simulink model "MSIP_Speed_Control_abc1a_84"  (R2025a)
settings: Solver=FixedStepAuto  StartTime=0.0  StopTime=150  FixedStep=1e-4  MaxStep=1e-3  RelTol=1e-3
model workspace (MAT data in the model file):
  Freq = 60
values from neighbouring files (symbols this model uses):
  b_MS = 1e-3    (= 0.001)    [data_MSIP_julio2025.m]
  beta_d_MS = pd_MS    (= 40)    [data_MSIP_julio2025.m]
  gamq = 2*J_MS*Lq_MS/(3*np_MS*lambda_MS)    (= 0.00452625826005)    [data_MSIP_julio2025.m]
  J_MS = 1e-1    (= 0.1)    [data_MSIP_julio2025.m]
  lambda_MS = 67.09e-2    (= 0.6709)    [data_MSIP_julio2025.m]
  Ld_MS = 22.1e-3    (= 0.0221)    [data_MSIP_julio2025.m]
  Lq_MS = 91.1e-3    (= 0.0911)    [data_MSIP_julio2025.m]
  np_MS = 2    [data_MSIP_julio2025.m]
  Rs_MS = 6.51e-1    (= 0.651)    [data_MSIP_julio2025.m]
undefined symbols (not defined in the file or in its folder): plecs
libraries: plecslib_extras2 x3, spsRMSLib x2, spsPLL3phLib x1, nesl_utility x1, spsTHDLib x1
(part 1 of 2)
settings Model: SimulationMode=accelerator  PauseTimes=0.01  Creator=RUBEN TAPIA OLVERA  LastModifiedBy=avalder
settings SolverCC: AlgebraicLoopSolver=TrustRegion
settings DataIOCC: ReturnWorkspaceOutputs=off
settings OptimizationCC: LifeSpan=inf
settings DebuggingCC: MaxConsecutiveZCsMsg=none  UnconnectedInputMsg=warning  UnconnectedOutputMsg=warning  UnconnectedLineMsg=warning  SFUnexpectedBacktrackingDiag=warning  SFNoUnconditionalDefaultTransitionDiag=warning  SFExecutionAtInitializationDiag=none  ArithmeticOperatorsInVariantConditions=warning
settings ModelReferenceCC: EnableRefExpFcnMdlSchedulingChecks=on
settings SFSimCC: SimUseLocalCustomCode=off  CustomCodeUndefinedFunction=UseInterfaceOnly
settings RTWCC: RTWUseLocalCustomCode=off  GPUComputeCapability=3.5
settings CodeAppCC: StateflowObjectComments=on
settings GRTTargetCC: TargetLangStandard=C89/C90 (ANSI)
settings ConfigComp: CovMetricSettings=dw  CovSaveCumulativeToWorkspaceVar=on  CovSaveSingleToWorkspaceVar=on  CovExternalEMLEnable=off
settings SimscapeCC: SimscapeNormalizeSystem=off

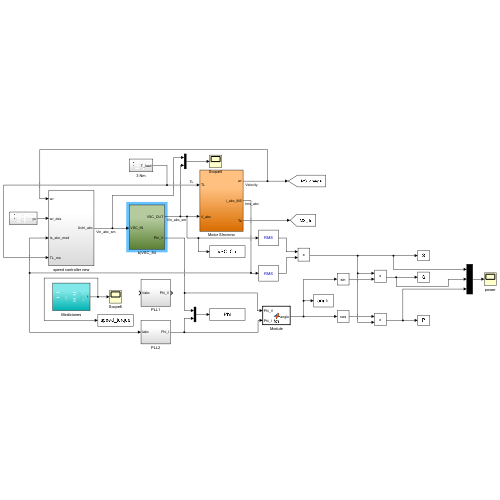
[thumbnail: Simulink's stored preview of the top-level diagram]
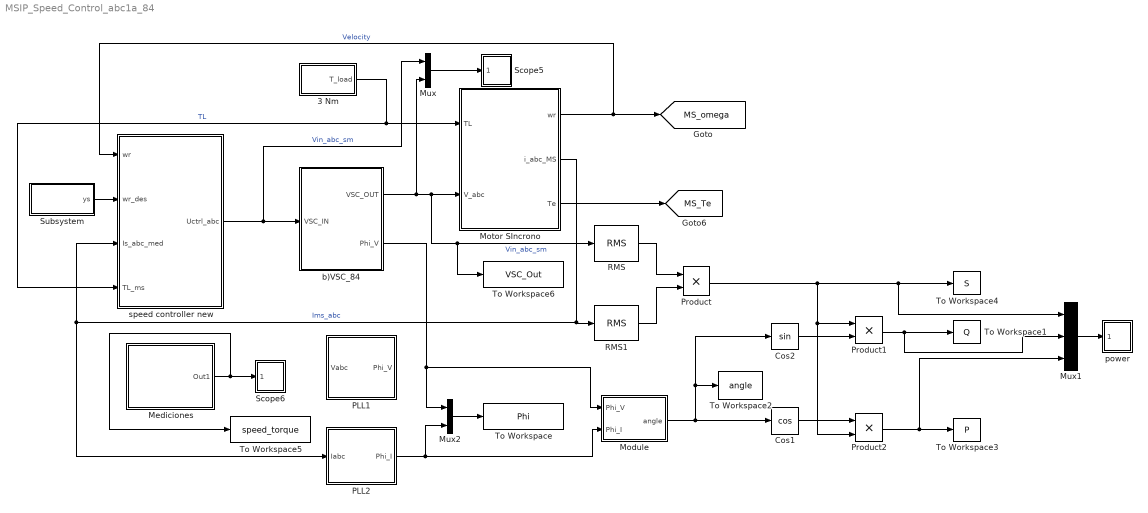
== system MSIP_Speed_Control_abc1a_84 ==
  3 Nm : Subsystem
  Cos1 : Trigonometry  Operator=cos
  Cos2 : Trigonometry
  Mediciones : Subsystem
  Module : MATLAB Function  TreatAsAtomicUnit=on
  Motor SIncrono : Subsystem
  Mux : Mux  Inputs=2
  Mux1 : Mux  Inputs=3
  Mux2 : Mux  Inputs=2
  PLL1 : Subsystem
  PLL2 : Subsystem
  Product : Product
  Product1 : Product
  Product2 : Product
  RMS : spsRMSLib/RMS  TrueRMS=on  Freq=Freq  RMSInit=0  Ts=0
  RMS1 : spsRMSLib/RMS  TrueRMS=on  Freq=Freq  RMSInit=0  Ts=0
  Scope5 : Subsystem  LoadFcn=plecs('sl', 300);  InitFcn=plecs('sl', 314);  StartFcn=plecs('sl', 308);  StopFcn=plecs('sl', 309);  mask{Settings=<binary blob, 776 chars, not shown>}
      mask init:
      | plecs('sl', 315);
      settings: CopyFcn=plecs('sl', 303);  DeleteFcn=plecs('sl', 305);  UndoDeleteFcn=plecs('sl', 306);  PreSaveFcn=plecs('sl', 311);  NameChangeFcn=plecs('sl', 310);  DestroyFcn=plecs('sl', 307);  OpenFcn=plecs('sl', 302);  ErrorFcn=plerrorfcn
      mask Display: plot([0.1 0.9 0.9 0.1 0.1], [0.9 0.9 0.5 0.5 0.9])
  Scope6 : Subsystem  LoadFcn=plecs('sl', 300);  InitFcn=plecs('sl', 314);  StartFcn=plecs('sl', 308);  StopFcn=plecs('sl', 309);  mask{Settings=<binary blob, 752 chars, not shown>}
      mask init:
      | plecs('sl', 315);
      settings: CopyFcn=plecs('sl', 303);  DeleteFcn=plecs('sl', 305);  UndoDeleteFcn=plecs('sl', 306);  PreSaveFcn=plecs('sl', 311);  NameChangeFcn=plecs('sl', 310);  DestroyFcn=plecs('sl', 307);  OpenFcn=plecs('sl', 302);  ErrorFcn=plerrorfcn
      mask Display: plot([0.1 0.9 0.9 0.1 0.1], [0.9 0.9 0.5 0.5 0.9])
  Subsystem : Subsystem
  To Workspace : ToWorkspace  VariableName=Phi  SaveFormat=Timeseries  SampleTime=-1
  To Workspace1 : ToWorkspace  VariableName=Q  SaveFormat=Timeseries  SampleTime=-1
  To Workspace2 : ToWorkspace  VariableName=angle  SaveFormat=Timeseries  SampleTime=-1
  To Workspace3 : ToWorkspace  VariableName=P  SaveFormat=Timeseries  SampleTime=-1
  To Workspace4 : ToWorkspace  VariableName=S  SaveFormat=Timeseries  SampleTime=-1
  To Workspace5 : ToWorkspace  VariableName=speed_torque  SaveFormat=Timeseries  SampleTime=-1
  To Workspace6 : ToWorkspace  VariableName=VSC_Out  SaveFormat=Timeseries  SampleTime=-1
  b)VSC_84 : Subsystem
  power : Subsystem  LoadFcn=plecs('sl', 300);  InitFcn=plecs('sl', 314);  StartFcn=plecs('sl', 308);  StopFcn=plecs('sl', 309);  mask{Settings=<binary blob, 756 chars, not shown>}
      mask init:
      | plecs('sl', 315);
      settings: CopyFcn=plecs('sl', 303);  DeleteFcn=plecs('sl', 305);  UndoDeleteFcn=plecs('sl', 306);  PreSaveFcn=plecs('sl', 311);  NameChangeFcn=plecs('sl', 310);  DestroyFcn=plecs('sl', 307);  OpenFcn=plecs('sl', 302);  ErrorFcn=plerrorfcn
      mask Display: plot([0.1 0.9 0.9 0.1 0.1], [0.9 0.9 0.5 0.5 0.9])
  speed controller new : Subsystem
  tag scope: MS_Te=global, MS_omega=global
  wires:
  Motor SIncrono/1(wr) -> speed controller new/1(wr), [MS_omega]  "Velocity"
  3 Nm/1(T_load) -> speed controller new/4(TL_ms), Motor SIncrono/1(TL)  "TL"
  Motor SIncrono/3(Te) -> [MS_Te]
  Motor SIncrono/2(i_abc_MS) -> RMS1/1, speed controller new/3(Is_abc_med), PLL2/1(Iabc)  "Ims_abc"
  Subsystem/1(ys) -> speed controller new/2(wr_des)
  Mux2/1 -> To Workspace/1
  Module/1(angle) -> Cos1/1, To Workspace2/1, Cos2/1
  b)VSC_84/1(VSC_OUT) -> Mux/2, Motor SIncrono/2(V_abc), To Workspace6/1, RMS/1  "Vin_abc_sm"
  b)VSC_84/2(Phi_V) -> Mux2/1, Module/1(Phi_V)
  PLL2/1(Phi_I) -> Module/2(Phi_I), Mux2/2
  speed controller new/1(Uctrl_abc) -> b)VSC_84/1(VSC_IN), Mux/1  "Vin_abc_sm"
  Product/1 -> Product2/2, Product1/1, Mux1/1, To Workspace4/1
  RMS/1 -> Product/1
  RMS1/1 -> Product/2
  Mux/1 -> Scope5/1(1)
  Mediciones/1(Out1) -> To Workspace5/1, Scope6/1(1)
  Cos2/1 -> Product1/2
  Cos1/1 -> Product2/1
  Product1/1 -> Mux1/2, To Workspace1/1
  Product2/1 -> Mux1/3, To Workspace3/1
  Mux1/1 -> power/1(1)

== system MSIP_Speed_Control_abc1a_84/3 Nm ==
  Add : Sum  Inputs=+++
  TL1 : MATLAB Function  TreatAsAtomicUnit=on
  TL2 : MATLAB Function  TreatAsAtomicUnit=on
  TL3 : MATLAB Function  TreatAsAtomicUnit=on
  Tiempo1 : Clock
  T_load : Outport
  tag scope: TL_MS=global
  wires:
  Tiempo1/1 -> TL3/1(t), TL2/1(t), TL1/1(t)
  TL3/1(T_load3) -> Add/3
  TL1/1(T_load) -> Add/1
  TL2/1(T_load2) -> Add/2
  Add/1 -> T_load/1, [TL_MS]

== system MSIP_Speed_Control_abc1a_84/Mediciones ==
  Demux : Demux  Outputs=2
  Mux : Mux  Inputs=2
  Mux1 : Mux  Inputs=2
  Mux2 : Mux  Inputs=2
  Scope{1,3..6} (5 alike) : Scope
      Scope1 settings: Title=Currents  ActiveDisplayYMinimum=-0.00105  ActiveDisplayYMaximum=0.01123  DataLoggingVariableName=ScopeData3
      Scope3 settings: ActiveDisplayYMinimum=-1  ActiveDisplayYMaximum=1
      Scope4 settings: ActiveDisplayYMinimum=-1  ActiveDisplayYMaximum=1  DataLoggingVariableName=ScopeData4
      Scope5 settings: Title=Currents  ActiveDisplayYMinimum=-0.003  ActiveDisplayYMaximum=0.00033
      Scope6 settings: ActiveDisplayYMinimum=-23.57031  ActiveDisplayYMaximum=212.1328
  Out1 : Outport
  wires:
  [MS_omega] -> Scope3/1
  [TL_MS] -> Mux2/1  "MI_TL"
  Mux2/1 -> Mux/2, Scope4/1
  [MS_Te] -> Mux2/2  "MI_Te"
  [Idq_MS] -> Demux/1
  Demux/1 -> Scope1/1
  Demux/2 -> Scope5/1
  [MS_omega] -> Mux1/2  "w"
  [MSIP_w_des] -> Mux1/1  "w_req"
  Mux1/1 -> Mux/1, Scope6/1
  Mux/1 -> Out1/1

== system MSIP_Speed_Control_abc1a_84/Motor SIncrono ==
  TL : Inport
  V_abc : Inport  Port=2
  Clock : Clock
  Clock1 : Clock
  Demux : Demux  Outputs=2
  Electrical Subsystem : Subsystem
  Mechanical Subsystem : Subsystem
  Mux2 : Mux  Inputs=2
  abc/dq : Subsystem
  dq/abc : Subsystem
  wr : Outport
  i_abc_MS : Outport  Port=2
  Te : Outport  Port=3
  tag scope: Idq_MS=global
  wires:
  Mechanical Subsystem/1(wr_MS) -> wr/1, Electrical Subsystem/1(w)
  TL/1 -> Mechanical Subsystem/1(TL)
  Mechanical Subsystem/2(Te_MS) -> Te/1
  Demux/1 -> Electrical Subsystem/2(U_d_MS)
  Demux/2 -> Electrical Subsystem/3(U_q_MS)
  Electrical Subsystem/1(id_MS) -> Mux2/1, Mechanical Subsystem/2(i_d_MS)  "id"
  Electrical Subsystem/2(iq_MS) -> Mechanical Subsystem/3(i_q_MS), Mux2/2  "iq"
  Mux2/1 -> dq/abc/2(Ud_m), [Idq_MS]  "i_dq"
  Clock/1 -> dq/abc/1(t)
  dq/abc/1(Uabc_m) -> i_abc_MS/1  "abc"
  Clock1/1 -> abc/dq/1(t)
  abc/dq/1(Udq_m) -> Demux/1  "a"
  V_abc/1 -> abc/dq/2(Uabc_m)

== system MSIP_Speed_Control_abc1a_84/PLL1 ==
  Vabc : Inport
  3ph->SRF : plecslib_extras2/Transformations/3ph->SRF
      settings: SourceProductName=PLECS Extras
  Constant1 : Constant  Value=pi/2
  Demux : Demux  Outputs=2
  Divide : Product  Inputs=/*
  Kp1 : Gain  Gain=-1  SaturateOnIntegerOverflow=on  OutDataTypeStr=Inherit: Same as input  ParamDataTypeStr=Inherit: Same as input
  Kp2 : Gain  Gain=2  SaturateOnIntegerOverflow=on  OutDataTypeStr=Inherit: Same as input  ParamDataTypeStr=Inherit: Same as input
  Module : MATLAB Function  TreatAsAtomicUnit=on
  Sum2 : Sum  Inputs=|+-
  Sum3 : Sum  Inputs=|++
  Trigonometric Function2 : Trigonometry  Operator=atan
  Phi_V : Outport
  wires:
  Demux/2 -> Divide/2
  Vabc/1 -> 3ph->SRF/1
  Demux/1 -> Sum2/2
  Sum2/1 -> Divide/1
  Divide/1 -> Trigonometric Function2/1
  Sum3/1 -> Kp2/1
  Module/1(y) -> Sum2/1
  Kp2/1 -> Phi_V/1
  Trigonometric Function2/1 -> Kp1/1
  Kp1/1 -> Sum3/1
  Constant1/1 -> Sum3/2
  3ph->SRF/1 -> Demux/1, Module/1(u)

== system MSIP_Speed_Control_abc1a_84/PLL2 ==
  Iabc : Inport
  3ph->SRF : plecslib_extras2/Transformations/3ph->SRF
      settings: SourceProductName=PLECS Extras
  Constant1 : Constant  Value=pi/2
  Demux : Demux  Outputs=2
  Divide : Product  Inputs=/*
  Kp1 : Gain  Gain=-1  SaturateOnIntegerOverflow=on  OutDataTypeStr=Inherit: Same as input  ParamDataTypeStr=Inherit: Same as input
  Kp2 : Gain  Gain=2  SaturateOnIntegerOverflow=on  OutDataTypeStr=Inherit: Same as input  ParamDataTypeStr=Inherit: Same as input
  Module : MATLAB Function  TreatAsAtomicUnit=on
  Sum2 : Sum  Inputs=|+-
  Sum3 : Sum  Inputs=|++
  Trigonometric Function2 : Trigonometry  Operator=atan
  Phi_I : Outport
  wires:
  Demux/2 -> Divide/2
  Iabc/1 -> 3ph->SRF/1
  Demux/1 -> Sum2/2
  Sum2/1 -> Divide/1
  Divide/1 -> Trigonometric Function2/1
  Sum3/1 -> Kp2/1
  Module/1(y) -> Sum2/1
  Kp2/1 -> Phi_I/1
  Trigonometric Function2/1 -> Kp1/1
  Kp1/1 -> Sum3/1
  Constant1/1 -> Sum3/2
  3ph->SRF/1 -> Demux/1, Module/1(u)

== system MSIP_Speed_Control_abc1a_84/Scope5 ==
  1 : Inport
  " InputMux " : Subsystem
      mask Display: disp('Mux')
  " S-Function " : S-Function  FunctionName=plecs  SFunctionDeploymentMode=off  EnableBusSupport=off
  wires:
  1/1 -> " InputMux "/1(In1)
  " InputMux "/1(Out) -> " S-Function "/1

== system MSIP_Speed_Control_abc1a_84/Scope6 ==
  1 : Inport
  " InputMux " : Subsystem
      mask Display: disp('Mux')
  " S-Function " : S-Function  FunctionName=plecs  SFunctionDeploymentMode=off  EnableBusSupport=off
  wires:
  1/1 -> " InputMux "/1(In1)
  " InputMux "/1(Out) -> " S-Function "/1

== system MSIP_Speed_Control_abc1a_84/Subsystem ==
  Add : Sum  Inputs=+++
  Theta_Deseada : MATLAB Function  TreatAsAtomicUnit=on
  Theta_Deseada1 : MATLAB Function  TreatAsAtomicUnit=on
  Theta_Deseada2 : MATLAB Function  TreatAsAtomicUnit=on
  Tiempo1 : Clock
  ys : Outport
  tag scope: MSIP_w_des=global
  wires:
  Tiempo1/1 -> Theta_Deseada1/1(t), Theta_Deseada2/1(t), Theta_Deseada/1(t)
  Theta_Deseada/1(ys) -> Add/1
  Theta_Deseada1/1(ys) -> Add/2
  Theta_Deseada2/1(ys) -> Add/3
  Add/1 -> ys/1, [MSIP_w_des]

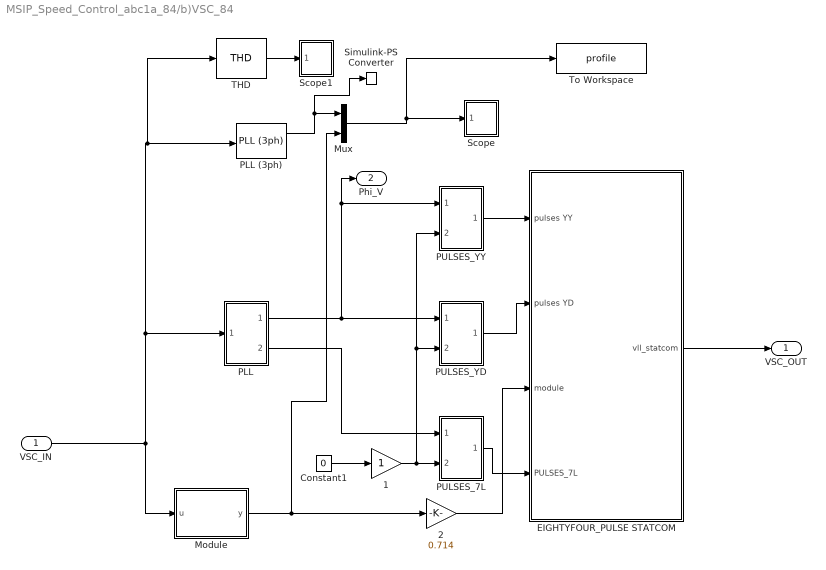
== system MSIP_Speed_Control_abc1a_84/b)VSC_84 ==
  VSC_IN : Inport
  1 : Gain  SaturateOnIntegerOverflow=on  OutDataTypeStr=Inherit: Same as input  ParamDataTypeStr=Inherit: Same as input
  2 : Gain  Gain=0.714  SaturateOnIntegerOverflow=on  OutDataTypeStr=Inherit: Same as input  ParamDataTypeStr=Inherit: Same as input
  Constant1 : Constant  Value=0
  EIGHTYFOUR_PULSE STATCOM : Subsystem  LoadFcn=plecs('sl', 200);  InitFcn=plecs('sl', 214);  StartFcn=plecs('sl', 208);  StopFcn=plecs('sl', 209);  mask(PlecsCircuit){PLECSData=<binary blob, 7880 chars, not shown>}
      mask prompts: PLECSData "PLECS Data (Do not delete or modify!)"
      mask help: Drag this block into a Simulink model to create a new electrical circuit.
      mask init:
      | % PLACE CUSTOM INITIALIZATIONS ABOVE
      | % DO NOT REMOVE
      | plecs('sl', 215);
      | % DO NOT REMOVE
      settings: CopyFcn=plecs('sl', 203);  DeleteFcn=plecs('sl', 205);  UndoDeleteFcn=plecs('sl', 206);  PreSaveFcn=plecs('sl', 211);  PostSaveFcn=plecs('sl', 201);  NameChangeFcn=plecs('sl', 210);  DestroyFcn=plecs('sl', 207);  PreCopyFcn=plecs('sl', 216);  OpenFcn=plecs('sl', 202);  ErrorFcn=plerrorfcn
      mask Display: disp('PLECS\nCircuit')
  Module : MATLAB Function  TreatAsAtomicUnit=on
  Mux : Mux  Inputs=2
  PLL : Subsystem
  PLL (3ph) : spsPLL3phLib/PLL (3ph)  Fmin=45  Par_Init=[0, 60]  ParK=[180, 3200, 1]  TcD=1e-4  MaxRateChangeFreq=12  FilterCutOffFreq=25  Ts=0  AGC=on
  PULSES_7L : Subsystem
  PULSES_YD : Subsystem
  PULSES_YY : Subsystem
  Scope : Subsystem  LoadFcn=plecs('sl', 300);  InitFcn=plecs('sl', 314);  StartFcn=plecs('sl', 308);  StopFcn=plecs('sl', 309);  mask{Settings=<binary blob, 752 chars, not shown>}
      mask init:
      | plecs('sl', 315);
      settings: CopyFcn=plecs('sl', 303);  DeleteFcn=plecs('sl', 305);  UndoDeleteFcn=plecs('sl', 306);  PreSaveFcn=plecs('sl', 311);  NameChangeFcn=plecs('sl', 310);  DestroyFcn=plecs('sl', 307);  OpenFcn=plecs('sl', 302);  ErrorFcn=plerrorfcn
      mask Display: plot([0.1 0.9 0.9 0.1 0.1], [0.9 0.9 0.5 0.5 0.9])
  Scope1 : Subsystem  LoadFcn=plecs('sl', 300);  InitFcn=plecs('sl', 314);  StartFcn=plecs('sl', 308);  StopFcn=plecs('sl', 309);  mask{Settings=<binary blob, 752 chars, not shown>}
      mask init:
      | plecs('sl', 315);
      settings: CopyFcn=plecs('sl', 303);  DeleteFcn=plecs('sl', 305);  UndoDeleteFcn=plecs('sl', 306);  PreSaveFcn=plecs('sl', 311);  NameChangeFcn=plecs('sl', 310);  DestroyFcn=plecs('sl', 307);  OpenFcn=plecs('sl', 302);  ErrorFcn=plerrorfcn
      mask Display: plot([0.1 0.9 0.9 0.1 0.1], [0.9 0.9 0.5 0.5 0.9])
  Simulink-PS Converter : nesl_utility/Simulink-PS Converter  PhysicalDomain=network_engine_domain  SubClassName=ps_input  LeftPortType=input  RightPortType=output  PseudoPeriodic=off  Frequencies=[]  NoiseDistribution=none  NoiseParameters=[]  Unit=1  AffineConversion=off  FilteringAndDerivatives=provide  SimscapeFilterOrder=1  InputFilterTimeConstant=0.001  UdotUserProvided=0
  THD : spsTHDLib/THD  Freq=Freq  Ts=0
  To Workspace : ToWorkspace  VariableName=profile  SaveFormat=Timeseries  SampleTime=-1
  VSC_OUT : Outport
  Phi_V : Outport  Port=2
  wires:
  PULSES_7L/1(pulses) -> EIGHTYFOUR_PULSE STATCOM/4(PULSES_7L)
  2/1 -> EIGHTYFOUR_PULSE STATCOM/3(module)
  Constant1/1 -> 1/1
  1/1 -> PULSES_7L/2(delta), PULSES_YD/2(delta), PULSES_YY/2(delta)
  PULSES_YY/1(pulses) -> EIGHTYFOUR_PULSE STATCOM/1(pulses YY)
  PULSES_YD/1(pulses) -> EIGHTYFOUR_PULSE STATCOM/2(pulses YD)
  EIGHTYFOUR_PULSE STATCOM/1(vll_statcom) -> VSC_OUT/1
  VSC_IN/1 -> THD/1, PLL (3ph)/1, PLL/1(In1), Module/1(u)
  PLL/1(phi) -> Phi_V/1, PULSES_YY/1(phi), PULSES_YD/1(phi)
  PLL/2(phi1) -> PULSES_7L/1(phi1)
  PLL (3ph)/1 -> Simulink-PS Converter/1, Mux/1
  Module/1(y) -> Mux/2, 2/1
  Mux/1 -> To Workspace/1, Scope/1(1)
  THD/1 -> Scope1/1(1)

== system MSIP_Speed_Control_abc1a_84/power ==
  1 : Inport
  " InputMux " : Subsystem
      mask Display: disp('Mux')
  " S-Function " : S-Function  FunctionName=plecs  SFunctionDeploymentMode=off  EnableBusSupport=off
  wires:
  1/1 -> " InputMux "/1(In1)
  " InputMux "/1(Out) -> " S-Function "/1

== system MSIP_Speed_Control_abc1a_84/speed controller new ==
  wr : Inport
  wr_des : Inport  Port=2
  Is_abc_med : Inport  Port=3
  TL_ms : Inport  Port=4
  Clock : Clock
  Mux : Mux  Inputs=2
  control loop U_wr : Subsystem
  dq/abc : Subsystem
  Uctrl_abc : Outport
  tag scope: Vin_MS=global
  wires:
  wr/1 -> control loop U_wr/2(wr)
  wr_des/1 -> control loop U_wr/1(wr_ref)
  TL_ms/1 -> control loop U_wr/4(TLms)
  Is_abc_med/1 -> control loop U_wr/3(Ims_abc)
  control loop U_wr/1(U1_d) -> Mux/1  "U_theta"
  control loop U_wr/2(U1_q) -> Mux/2
  Clock/1 -> dq/abc/1(t)
  Mux/1 -> dq/abc/2(Ud_m), [Vin_MS]  "i_dq"
  dq/abc/1(Uabc_m) -> Uctrl_abc/1  "abc"

== system MSIP_Speed_Control_abc1a_84/Motor SIncrono/Electrical Subsystem ==
  w : Inport
  U_d_MS : Inport  Port=2
  U_q_MS : Inport  Port=3
  Currents : Subsystem
  id_MS : Outport
  iq_MS : Outport  Port=2
  wires:
  w/1 -> Currents/1(w)
  Currents/1(id_Msinc) -> id_MS/1
  Currents/2(iq_Msinc) -> iq_MS/1
  U_d_MS/1 -> Currents/2(UdMS)
  U_q_MS/1 -> Currents/3(UqMS)

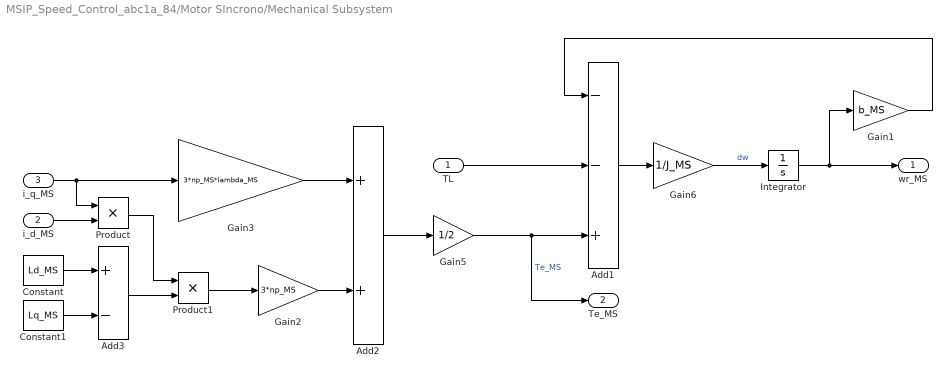
== system MSIP_Speed_Control_abc1a_84/Motor SIncrono/Mechanical Subsystem ==
  TL : Inport
  i_d_MS : Inport  Port=2
  i_q_MS : Inport  Port=3
  Add1 : Sum  Inputs=--+
  Add2 : Sum
  Add3 : Sum  Inputs=+-
  Constant : Constant  Value=Ld_MS
  Constant1 : Constant  Value=Lq_MS
  Gain1 : Gain  Gain=b_MS
  Gain2 : Gain  Gain=3*np_MS
  Gain3 : Gain  Gain=3*np_MS*lambda_MS
  Gain5 : Gain  Gain=1/2
  Gain6 : Gain  Gain=1/J_MS
  Integrator : Integrator
  Product : Product
  Product1 : Product
  wr_MS : Outport
  Te_MS : Outport  Port=2
  wires:
  Gain5/1 -> Te_MS/1, Add1/3  "Te_MS"
  Gain2/1 -> Add2/2
  TL/1 -> Add1/2
  i_d_MS/1 -> Product/2
  Product1/1 -> Gain2/1
  Gain3/1 -> Add2/1
  Gain1/1 -> Add1/1
  Add3/1 -> Product1/2
  Product/1 -> Product1/1
  Constant1/1 -> Add3/2
  Constant/1 -> Add3/1
  i_q_MS/1 -> Product/1, Gain3/1
  Add2/1 -> Gain5/1
  Integrator/1 -> wr_MS/1, Gain1/1
  Add1/1 -> Gain6/1
  Gain6/1 -> Integrator/1  "dw"

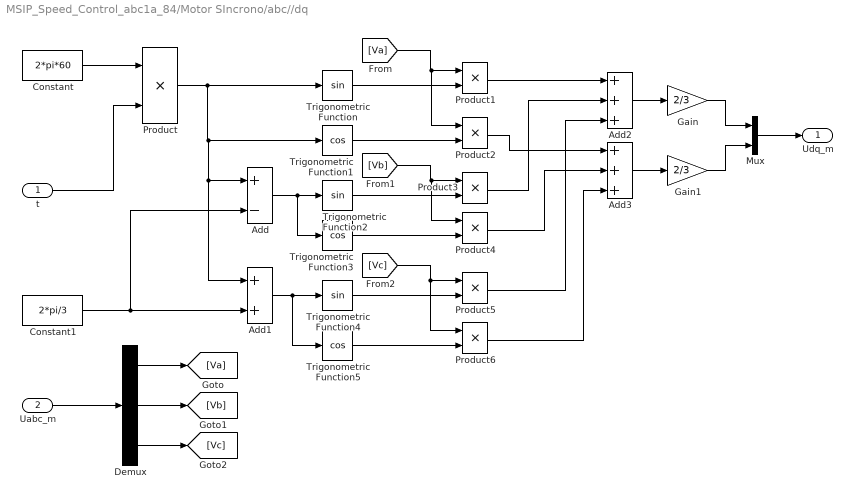
== system MSIP_Speed_Control_abc1a_84/Motor SIncrono/abc//dq ==
  t : Inport
  Uabc_m : Inport  Port=2
  Add : Sum  Inputs=+-
  Add1 : Sum
  Add2 : Sum  Inputs=+++
  Add3 : Sum  Inputs=+++
  Constant : Constant  Value=2*pi*60
  Constant1 : Constant  Value=2*pi/3
  Demux : Demux  Outputs=3
  Gain : Gain  Gain=2/3
  Gain1 : Gain  Gain=2/3
  Mux : Mux  Inputs=2
  Product{,1..6} (7 alike) : Product
  Trigonometric Function : Trigonometry
  Trigonometric Function1 : Trigonometry  Operator=cos
  Trigonometric Function2 : Trigonometry
  Trigonometric Function3 : Trigonometry  Operator=cos
  Trigonometric Function4 : Trigonometry
  Trigonometric Function5 : Trigonometry  Operator=cos
  Udq_m : Outport
  wires:
  t/1 -> Product/2
  Constant/1 -> Product/1
  Product/1 -> Add1/1, Add/1, Trigonometric Function1/1, Trigonometric Function/1
  Constant1/1 -> Add1/2, Add/2
  Add/1 -> Trigonometric Function3/1, Trigonometric Function2/1
  Add1/1 -> Trigonometric Function5/1, Trigonometric Function4/1
  Trigonometric Function/1 -> Product1/2
  Trigonometric Function2/1 -> Product3/2
  Uabc_m/1 -> Demux/1
  Add2/1 -> Gain/1
  Add3/1 -> Gain1/1
  Demux/1 -> [Va]
  Demux/2 -> [Vb]
  Demux/3 -> [Vc]
  [Va] -> Product2/1, Product1/1
  Product1/1 -> Add2/1
  [Vb] -> Product4/1, Product3/1
  Product3/1 -> Add2/2
  Trigonometric Function4/1 -> Product5/2
  [Vc] -> Product6/1, Product5/1
  Product5/1 -> Add2/3
  Product2/1 -> Add3/1
  Trigonometric Function5/1 -> Product6/2
  Trigonometric Function3/1 -> Product4/2
  Trigonometric Function1/1 -> Product2/2
  Product4/1 -> Add3/2
  Product6/1 -> Add3/3
  Mux/1 -> Udq_m/1
  Gain/1 -> Mux/1
  Gain1/1 -> Mux/2

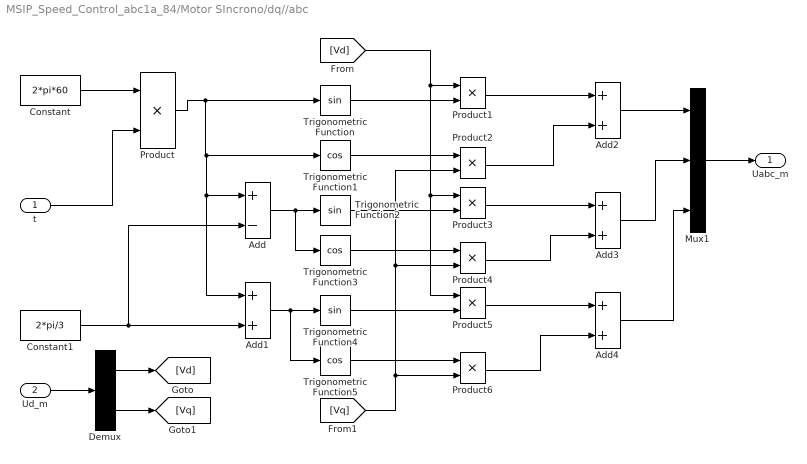
== system MSIP_Speed_Control_abc1a_84/Motor SIncrono/dq//abc ==
  t : Inport
  Ud_m : Inport  Port=2
  Add : Sum  Inputs=+-
  Add{1..4} (4 alike) : Sum
  Constant : Constant  Value=2*pi*60
  Constant1 : Constant  Value=2*pi/3
  Demux : Demux  Outputs=2
  Mux1 : Mux  Inputs=3
  Product{,1..6} (7 alike) : Product
  Trigonometric Function : Trigonometry
  Trigonometric Function1 : Trigonometry  Operator=cos
  Trigonometric Function2 : Trigonometry
  Trigonometric Function3 : Trigonometry  Operator=cos
  Trigonometric Function4 : Trigonometry
  Trigonometric Function5 : Trigonometry  Operator=cos
  Uabc_m : Outport
  wires:
  t/1 -> Product/2
  Constant/1 -> Product/1
  Product/1 -> Add1/1, Add/1, Trigonometric Function1/1, Trigonometric Function/1
  Constant1/1 -> Add1/2, Add/2
  Add/1 -> Trigonometric Function3/1, Trigonometric Function2/1
  Add1/1 -> Trigonometric Function5/1, Trigonometric Function4/1
  Trigonometric Function/1 -> Product1/2
  Trigonometric Function1/1 -> Product2/1
  Product1/1 -> Add2/1
  Product2/1 -> Add2/2
  Trigonometric Function2/1 -> Product3/2
  Trigonometric Function3/1 -> Product4/1
  Product3/1 -> Add3/1
  Product4/1 -> Add3/2
  Trigonometric Function4/1 -> Product5/2
  Trigonometric Function5/1 -> Product6/1
  Product5/1 -> Add4/1
  Product6/1 -> Add4/2
  Mux1/1 -> Uabc_m/1
  Add2/1 -> Mux1/1
  Add3/1 -> Mux1/2
  Add4/1 -> Mux1/3
  Ud_m/1 -> Demux/1
  Demux/1 -> [Vd]
  Demux/2 -> [Vq]
  [Vd] -> Product5/1, Product3/1, Product1/1
  [Vq] -> Product4/2, Product2/2, Product6/2

== system MSIP_Speed_Control_abc1a_84/Scope5/ InputMux  ==
  In1 : Inport
  Convert1 : DataTypeConversion
  Mux : Mux  Inputs=1
  Out : Outport
  wires:
  Convert1/1 -> Mux/1
  In1/1 -> Convert1/1
  Mux/1 -> Out/1

== system MSIP_Speed_Control_abc1a_84/Scope6/ InputMux  ==
  In1 : Inport
  Convert1 : DataTypeConversion
  Mux : Mux  Inputs=1
  Out : Outport
  wires:
  Convert1/1 -> Mux/1
  In1/1 -> Convert1/1
  Mux/1 -> Out/1

== system MSIP_Speed_Control_abc1a_84/b)VSC_84/EIGHTYFOUR_PULSE STATCOM ==
  pulses YY : Inport  PortDimensions=6
  pulses YD : Inport  Port=2  PortDimensions=6
  module : Inport  Port=3  PortDimensions=1
  PULSES_7L : Inport  Port=4  PortDimensions=8
  " CircuitID48 " : Subsystem
  " GateMux " : Mux  Inputs=[ 6 6 8 ]
  " InputMux " : Mux  Inputs=[ 1 ]
  " OutputDemux " : Demux  Outputs=[ 3 ]
  " PULSES_7L " : DataTypeConversion
  " ProbeDemux " : Terminator
  " S-Function " : S-Function  FunctionName=plecs  SFunctionDeploymentMode=off  EnableBusSupport=off
  " module " : DataTypeConversion
  " pulses YD " : DataTypeConversion
  " pulses YY " : DataTypeConversion
  vll_statcom : Outport  PortDimensions=3
  wires:
  " InputMux "/1 -> " S-Function "/1
  " GateMux "/1 -> " S-Function "/2
  " S-Function "/1 -> " OutputDemux "/1
  " S-Function "/2 -> " ProbeDemux "/1
  module/1 -> " module "/1
  " module "/1 -> " InputMux "/1
  pulses YY/1 -> " pulses YY "/1
  " pulses YY "/1 -> " GateMux "/1
  pulses YD/1 -> " pulses YD "/1
  " pulses YD "/1 -> " GateMux "/2
  PULSES_7L/1 -> " PULSES_7L "/1
  " PULSES_7L "/1 -> " GateMux "/3
  " OutputDemux "/1 -> vll_statcom/1

== system MSIP_Speed_Control_abc1a_84/b)VSC_84/PLL ==
  In1 : Inport
  3ph->SRF : plecslib_extras2/Transformations/3ph->SRF
      settings: SourceProductName=PLECS Extras
  Constant1 : Constant  Value=pi/2
  Demux : Demux  Outputs=2
  Divide : Product  Inputs=/*
  Kp1 : Gain  Gain=-1  SaturateOnIntegerOverflow=on  OutDataTypeStr=Inherit: Same as input  ParamDataTypeStr=Inherit: Same as input
  Kp2 : Gain  Gain=2  SaturateOnIntegerOverflow=on  OutDataTypeStr=Inherit: Same as input  ParamDataTypeStr=Inherit: Same as input
  Math Function1 : Math  Operator=mod  SignedPower=on
  Module : MATLAB Function  TreatAsAtomicUnit=on
  Scope : Subsystem  LoadFcn=plecs('sl', 300);  InitFcn=plecs('sl', 314);  StartFcn=plecs('sl', 308);  StopFcn=plecs('sl', 309);  mask{Settings=<binary blob, 752 chars, not shown>}
      mask init:
      | plecs('sl', 315);
      settings: CopyFcn=plecs('sl', 303);  DeleteFcn=plecs('sl', 305);  UndoDeleteFcn=plecs('sl', 306);  PreSaveFcn=plecs('sl', 311);  NameChangeFcn=plecs('sl', 310);  DestroyFcn=plecs('sl', 307);  OpenFcn=plecs('sl', 302);  ErrorFcn=plerrorfcn
      mask Display: plot([0.1 0.9 0.9 0.1 0.1], [0.9 0.9 0.5 0.5 0.9])
  Sum2 : Sum  Inputs=|+-
  Sum3 : Sum  Inputs=|++
  Trigonometric Function2 : Trigonometry  Operator=atan
  w4 : Constant  Value=pi/3
  phi : Outport
  phi1 : Outport  Port=2
  wires:
  Math Function1/1 -> phi1/1
  w4/1 -> Math Function1/2
  Demux/2 -> Divide/2
  In1/1 -> 3ph->SRF/1
  Demux/1 -> Sum2/2
  Sum2/1 -> Divide/1
  Divide/1 -> Trigonometric Function2/1
  Sum3/1 -> Kp2/1
  Module/1(y) -> Sum2/1, Scope/1(1)
  Kp2/1 -> phi/1, Math Function1/1
  Trigonometric Function2/1 -> Kp1/1
  Kp1/1 -> Sum3/1
  Constant1/1 -> Sum3/2
  3ph->SRF/1 -> Demux/1, Module/1(u)

== system MSIP_Speed_Control_abc1a_84/b)VSC_84/PULSES_7L ==
  note: pi/3
  phi1 : Inport  PortDimensions=1
  delta : Inport  Port=2  PortDimensions=1
  MATLAB Function : MATLAB Function  TreatAsAtomicUnit=on
  Math Function1 : Math  Operator=mod  SignedPower=on
  Mux : Mux  Inputs=8
  Sum1 : Sum  InputSameDT=on  SaturateOnIntegerOverflow=on  OutDataTypeStr=Inherit: Same as first input
  w4 : Constant  Value=1.0472
  pulses : Outport
  wires:
  Math Function1/1 -> MATLAB Function/1(u)
  Mux/1 -> pulses/1
  MATLAB Function/8(s8) -> Mux/8
  MATLAB Function/7(s7) -> Mux/7
  MATLAB Function/6(s6) -> Mux/6
  MATLAB Function/5(s5) -> Mux/5
  MATLAB Function/4(s4) -> Mux/4
  MATLAB Function/3(s3) -> Mux/3
  MATLAB Function/2(s2) -> Mux/2
  MATLAB Function/1(s1) -> Mux/1
  phi1/1 -> Sum1/1
  delta/1 -> Sum1/2
  Sum1/1 -> Math Function1/1
  w4/1 -> Math Function1/2

== system MSIP_Speed_Control_abc1a_84/b)VSC_84/PULSES_YD ==
  note: -pi/6+pi/3
  note: 2pi
  phi : Inport  PortDimensions=1
  delta : Inport  Port=2  PortDimensions=1
  MATLAB Function : MATLAB Function  TreatAsAtomicUnit=on
  Math Function1 : Math  Operator=mod  SignedPower=on
  Mux : Mux  Inputs=6
  Sum1 : Sum  Inputs=+++  InputSameDT=on  SaturateOnIntegerOverflow=on  OutDataTypeStr=Inherit: Same as first input
  w1 : Constant  Value=0.5236
  w13 : Constant  Value=6.2832
  pulses : Outport
  wires:
  w1/1 -> Sum1/3
  Math Function1/1 -> MATLAB Function/1(u)
  Mux/1 -> pulses/1
  MATLAB Function/6(s6) -> Mux/6
  MATLAB Function/5(s5) -> Mux/5
  MATLAB Function/4(s4) -> Mux/4
  MATLAB Function/3(s3) -> Mux/3
  MATLAB Function/2(s2) -> Mux/2
  MATLAB Function/1(s1) -> Mux/1
  phi/1 -> Sum1/1
  delta/1 -> Sum1/2
  Sum1/1 -> Math Function1/1
  w13/1 -> Math Function1/2

== system MSIP_Speed_Control_abc1a_84/b)VSC_84/PULSES_YY ==
  note: 0+pi/3
  note: 2pi
  phi : Inport  PortDimensions=1
  delta : Inport  Port=2  PortDimensions=1
  MATLAB Function : MATLAB Function  TreatAsAtomicUnit=on
  Math Function1 : Math  Operator=mod  SignedPower=on
  Mux : Mux  Inputs=6
  Sum1 : Sum  Inputs=+++  InputSameDT=on  SaturateOnIntegerOverflow=on  OutDataTypeStr=Inherit: Same as first input
  w1 : Constant  Value=1.0472
  w2 : Constant  Value=6.2832
  pulses : Outport
  wires:
  w1/1 -> Sum1/3
  phi/1 -> Sum1/1
  delta/1 -> Sum1/2
  w2/1 -> Math Function1/2
  Sum1/1 -> Math Function1/1
  MATLAB Function/1(s1) -> Mux/1
  MATLAB Function/2(s2) -> Mux/2
  MATLAB Function/3(s3) -> Mux/3
  MATLAB Function/4(s4) -> Mux/4
  MATLAB Function/5(s5) -> Mux/5
  MATLAB Function/6(s6) -> Mux/6
  Mux/1 -> pulses/1
  Math Function1/1 -> MATLAB Function/1(u)

== system MSIP_Speed_Control_abc1a_84/b)VSC_84/Scope ==
  1 : Inport
  " InputMux " : Subsystem
      mask Display: disp('Mux')
  " S-Function " : S-Function  FunctionName=plecs  SFunctionDeploymentMode=off  EnableBusSupport=off
  wires:
  1/1 -> " InputMux "/1(In1)
  " InputMux "/1(Out) -> " S-Function "/1

== system MSIP_Speed_Control_abc1a_84/b)VSC_84/Scope1 ==
  1 : Inport
  " InputMux " : Subsystem
      mask Display: disp('Mux')
  " S-Function " : S-Function  FunctionName=plecs  SFunctionDeploymentMode=off  EnableBusSupport=off
  wires:
  1/1 -> " InputMux "/1(In1)
  " InputMux "/1(Out) -> " S-Function "/1

== system MSIP_Speed_Control_abc1a_84/power/ InputMux  ==
  In1 : Inport
  Convert1 : DataTypeConversion
  Mux : Mux  Inputs=1
  Out : Outport
  wires:
  Convert1/1 -> Mux/1
  In1/1 -> Convert1/1
  Mux/1 -> Out/1

== system MSIP_Speed_Control_abc1a_84/speed controller new/control loop U_wr ==
  wr_ref : Inport
  wr : Inport  Port=2
  Ims_abc : Inport  Port=3
  TLms : Inport  Port=4
  Clock : Clock
  Ctrl unit U1_d : Subsystem
  Ctrl unit U1_d1 : Subsystem
  abc/dq : Subsystem
  U1_d : Outport
  U1_q : Outport  Port=2
  wires:
  wr/1 -> Ctrl unit U1_d1/2(wr), Ctrl unit U1_d/1(wr)
  TLms/1 -> Ctrl unit U1_d1/3(MS_TL)
  Ims_abc/1 -> abc/dq/2(Uabc_m)
  Clock/1 -> abc/dq/1(t)
  abc/dq/1(Udq_m) -> Ctrl unit U1_d/2(MS_Idq)  "a"
  Ctrl unit U1_d/1(ud) -> U1_d/1
  Ctrl unit U1_d1/1(uq) -> U1_q/1
  wr_ref/1 -> Ctrl unit U1_d1/1(MSwr_des)

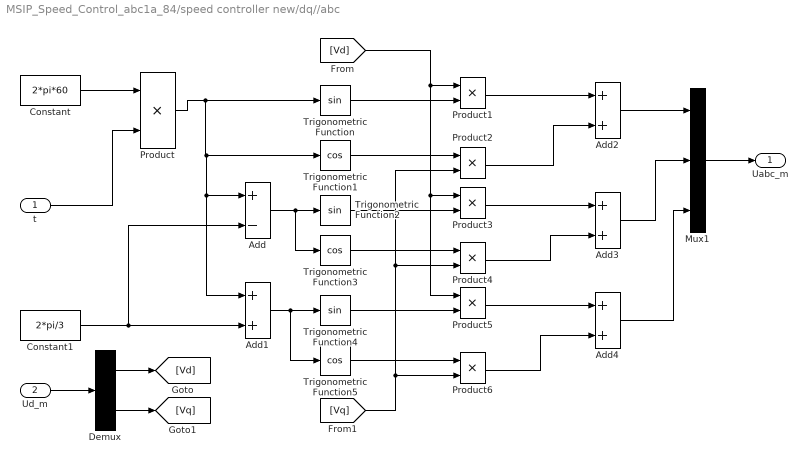
== system MSIP_Speed_Control_abc1a_84/speed controller new/dq//abc ==
  t : Inport
  Ud_m : Inport  Port=2
  Add : Sum  Inputs=+-
  Add{1..4} (4 alike) : Sum
  Constant : Constant  Value=2*pi*60
  Constant1 : Constant  Value=2*pi/3
  Demux : Demux  Outputs=2
  Mux1 : Mux  Inputs=3
  Product{,1..6} (7 alike) : Product
  Trigonometric Function : Trigonometry
  Trigonometric Function1 : Trigonometry  Operator=cos
  Trigonometric Function2 : Trigonometry
  Trigonometric Function3 : Trigonometry  Operator=cos
  Trigonometric Function4 : Trigonometry
  Trigonometric Function5 : Trigonometry  Operator=cos
  Uabc_m : Outport
  wires:
  t/1 -> Product/2
  Constant/1 -> Product/1
  Product/1 -> Add1/1, Add/1, Trigonometric Function1/1, Trigonometric Function/1
  Constant1/1 -> Add1/2, Add/2
  Add/1 -> Trigonometric Function3/1, Trigonometric Function2/1
  Add1/1 -> Trigonometric Function5/1, Trigonometric Function4/1
  Trigonometric Function/1 -> Product1/2
  Trigonometric Function1/1 -> Product2/1
  Product1/1 -> Add2/1
  Product2/1 -> Add2/2
  Trigonometric Function2/1 -> Product3/2
  Trigonometric Function3/1 -> Product4/1
  Product3/1 -> Add3/1
  Product4/1 -> Add3/2
  Trigonometric Function4/1 -> Product5/2
  Trigonometric Function5/1 -> Product6/1
  Product5/1 -> Add4/1
  Product6/1 -> Add4/2
  Mux1/1 -> Uabc_m/1
  Add2/1 -> Mux1/1
  Add3/1 -> Mux1/2
  Add4/1 -> Mux1/3
  Ud_m/1 -> Demux/1
  Demux/1 -> [Vd]
  Demux/2 -> [Vq]
  [Vd] -> Product5/1, Product3/1, Product1/1
  [Vq] -> Product4/2, Product2/2, Product6/2

== system MSIP_Speed_Control_abc1a_84/Motor SIncrono/Electrical Subsystem/Currents ==
  w : Inport
  UdMS : Inport  Port=2
  UqMS : Inport  Port=3
  Subsystem : Subsystem
  Subsystem1 : Subsystem
  id_Msinc : Outport
  iq_Msinc : Outport  Port=2
  wires:
  w/1 -> Subsystem1/1(wrMS), Subsystem/1(wrMS)
  UdMS/1 -> Subsystem/2(udMS)
  Subsystem/1(idMS) -> Subsystem1/3(idMS), id_Msinc/1
  Subsystem1/1(iq_Msinc) -> Subsystem/3(iqMS), iq_Msinc/1
  UqMS/1 -> Subsystem1/2(uqMS)

== system MSIP_Speed_Control_abc1a_84/b)VSC_84/EIGHTYFOUR_PULSE STATCOM/ CircuitID48  ==

== system MSIP_Speed_Control_abc1a_84/b)VSC_84/PLL/Scope ==
  1 : Inport
  " InputMux " : Subsystem
      mask Display: disp('Mux')
  " S-Function " : S-Function  FunctionName=plecs  SFunctionDeploymentMode=off  EnableBusSupport=off
  wires:
  " InputMux "/1(Out) -> " S-Function "/1
  1/1 -> " InputMux "/1(In1)

== system MSIP_Speed_Control_abc1a_84/b)VSC_84/Scope/ InputMux  ==
  In1 : Inport
  Convert1 : DataTypeConversion
  Mux : Mux  Inputs=1
  Out : Outport
  wires:
  Convert1/1 -> Mux/1
  In1/1 -> Convert1/1
  Mux/1 -> Out/1

== system MSIP_Speed_Control_abc1a_84/b)VSC_84/Scope1/ InputMux  ==
  In1 : Inport
  Convert1 : DataTypeConversion
  Mux : Mux  Inputs=1
  Out : Outport
  wires:
  Convert1/1 -> Mux/1
  In1/1 -> Convert1/1
  Mux/1 -> Out/1

== system MSIP_Speed_Control_abc1a_84/speed controller new/control loop U_wr/Ctrl unit U1_d ==
  wr : Inport
  MS_Idq : Inport  Port=2
  Add1 : Sum  Inputs=--
  Demux : Demux  Outputs=2
  Gain1 : Gain  Gain=beta_d_MS
  Gain2 : Gain  Gain=Lq_MS*np_MS
  Product : Product
  ud : Outport
  wires:
  Add1/1 -> ud/1
  MS_Idq/1 -> Demux/1
  Demux/1 -> Gain1/1  "Id"
  Demux/2 -> Product/2  "Iq"
  Gain1/1 -> Add1/1
  wr/1 -> Product/1
  Product/1 -> Gain2/1
  Gain2/1 -> Add1/2

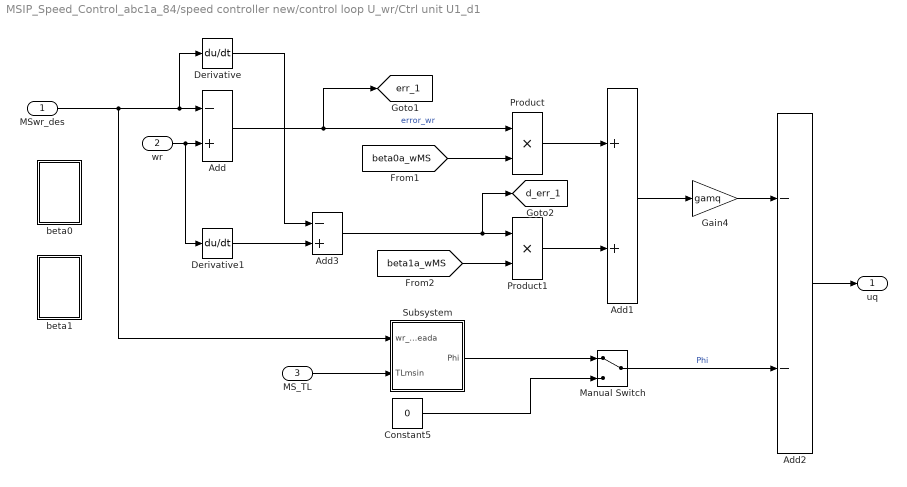
== system MSIP_Speed_Control_abc1a_84/speed controller new/control loop U_wr/Ctrl unit U1_d1 ==
  MSwr_des : Inport
  wr : Inport  Port=2
  MS_TL : Inport  Port=3
  Add : Sum  Inputs=-+
  Add1 : Sum
  Add2 : Sum  Inputs=--
  Add3 : Sum  Inputs=-+
  Constant5 : Constant  Value=0
  Derivative : Derivative
  Derivative1 : Derivative
  Gain4 : Gain  Gain=gamq
  Manual Switch : ManualSwitch
  Product : Product
  Product1 : Product
  Subsystem : Subsystem
  beta0 : Subsystem
  beta1 : Subsystem
  uq : Outport
  tag scope: d_err_1=global, err_1=global
  wires:
  MSwr_des/1 -> Subsystem/1(wr_deseada), Derivative/1, Add/1
  wr/1 -> Derivative1/1, Add/2
  Constant5/1 -> Manual Switch/2
  Manual Switch/1 -> Add2/2  "Phi"
  Add/1 -> Product/1, [err_1]  "error_wr"
  Product1/1 -> Add1/2
  Product/1 -> Add1/1
  MS_TL/1 -> Subsystem/2(TLmsin)
  Add3/1 -> [d_err_1], Product1/1
  Derivative/1 -> Add3/1
  Add2/1 -> uq/1
  Add1/1 -> Gain4/1
  Gain4/1 -> Add2/1
  Derivative1/1 -> Add3/2
  Subsystem/1(Phi) -> Manual Switch/1
  [beta0a_wMS] -> Product/2
  [beta1a_wMS] -> Product1/2

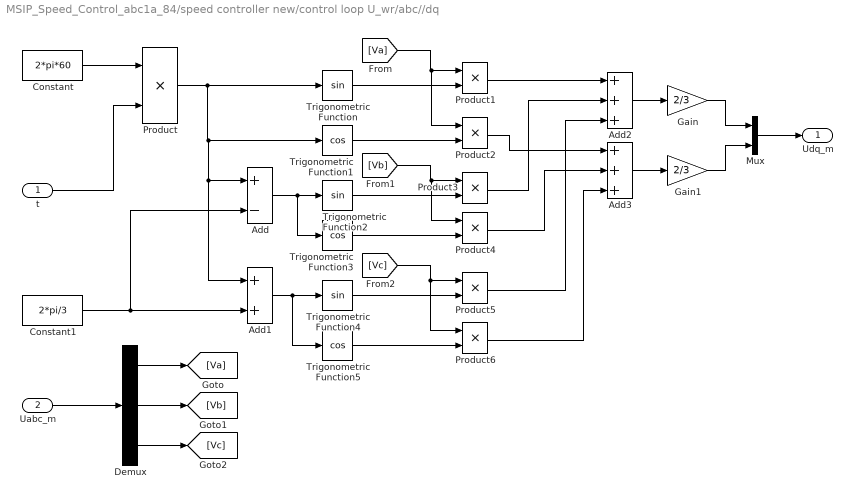
== system MSIP_Speed_Control_abc1a_84/speed controller new/control loop U_wr/abc//dq ==
  t : Inport
  Uabc_m : Inport  Port=2
  Add : Sum  Inputs=+-
  Add1 : Sum
  Add2 : Sum  Inputs=+++
  Add3 : Sum  Inputs=+++
  Constant : Constant  Value=2*pi*60
  Constant1 : Constant  Value=2*pi/3
  Demux : Demux  Outputs=3
  Gain : Gain  Gain=2/3
  Gain1 : Gain  Gain=2/3
  Mux : Mux  Inputs=2
  Product{,1..6} (7 alike) : Product
  Trigonometric Function : Trigonometry
  Trigonometric Function1 : Trigonometry  Operator=cos
  Trigonometric Function2 : Trigonometry
  Trigonometric Function3 : Trigonometry  Operator=cos
  Trigonometric Function4 : Trigonometry
  Trigonometric Function5 : Trigonometry  Operator=cos
  Udq_m : Outport
  wires:
  t/1 -> Product/2
  Constant/1 -> Product/1
  Product/1 -> Add1/1, Add/1, Trigonometric Function1/1, Trigonometric Function/1
  Constant1/1 -> Add1/2, Add/2
  Add/1 -> Trigonometric Function3/1, Trigonometric Function2/1
  Add1/1 -> Trigonometric Function5/1, Trigonometric Function4/1
  Trigonometric Function/1 -> Product1/2
  Trigonometric Function2/1 -> Product3/2
  Uabc_m/1 -> Demux/1
  Add2/1 -> Gain/1
  Add3/1 -> Gain1/1
  Demux/1 -> [Va]
  Demux/2 -> [Vb]
  Demux/3 -> [Vc]
  [Va] -> Product2/1, Product1/1
  Product1/1 -> Add2/1
  [Vb] -> Product4/1, Product3/1
  Product3/1 -> Add2/2
  Trigonometric Function4/1 -> Product5/2
  [Vc] -> Product6/1, Product5/1
  Product5/1 -> Add2/3
  Product2/1 -> Add3/1
  Trigonometric Function5/1 -> Product6/2
  Trigonometric Function3/1 -> Product4/2
  Trigonometric Function1/1 -> Product2/2
  Product4/1 -> Add3/2
  Product6/1 -> Add3/3
  Mux/1 -> Udq_m/1
  Gain/1 -> Mux/1
  Gain1/1 -> Mux/2

== system MSIP_Speed_Control_abc1a_84/Motor SIncrono/Electrical Subsystem/Currents/Subsystem ==
  wrMS : Inport
  udMS : Inport  Port=2
  iqMS : Inport  Port=3
  Add4 : Sum  Inputs=-++
  Gain1 : Gain  Gain=1/Ld_MS
  Gain2 : Gain  Gain=Rs_MS
  Gain3 : Gain  Gain=np_MS*Lq_MS
  Integrator3 : Integrator  InitialCondition=0.01
  Product2 : Product
  idMS : Outport
  wires:
  Integrator3/1 -> Gain2/1, idMS/1
  Gain1/1 -> Integrator3/1
  Add4/1 -> Gain1/1
  Gain2/1 -> Add4/1
  Gain3/1 -> Add4/2
  Product2/1 -> Gain3/1
  wrMS/1 -> Product2/1
  iqMS/1 -> Product2/2
  udMS/1 -> Add4/3

== system MSIP_Speed_Control_abc1a_84/Motor SIncrono/Electrical Subsystem/Currents/Subsystem1 ==
  wrMS : Inport
  uqMS : Inport  Port=2
  idMS : Inport  Port=3
  Add4 : Sum  Inputs=---+
  Gain1 : Gain  Gain=1/Lq_MS
  Gain2 : Gain  Gain=Rs_MS
  Gain3 : Gain  Gain=np_MS*Ld_MS
  Gain4 : Gain  Gain=np_MS*lambda_MS
  Integrator3 : Integrator
  Product2 : Product
  iq_Msinc : Outport
  wires:
  Product2/1 -> Gain3/1
  Gain3/1 -> Add4/2
  Gain2/1 -> Add4/1
  Add4/1 -> Gain1/1
  Gain1/1 -> Integrator3/1
  Integrator3/1 -> iq_Msinc/1, Gain2/1
  uqMS/1 -> Add4/4
  Gain4/1 -> Add4/3
  wrMS/1 -> Gain4/1, Product2/2
  idMS/1 -> Product2/1

== system MSIP_Speed_Control_abc1a_84/b)VSC_84/PLL/Scope/ InputMux  ==
  In1 : Inport
  Convert1 : DataTypeConversion
  Mux : Mux  Inputs=1
  Out : Outport
  wires:
  Mux/1 -> Out/1
  In1/1 -> Convert1/1
  Convert1/1 -> Mux/1

== system MSIP_Speed_Control_abc1a_84/speed controller new/control loop U_wr/Ctrl unit U1_d1/Subsystem ==
  wr_deseada : Inport
  TLmsin : Inport  Port=2
  Add : Sum  Inputs=----
  Add1 : Sum
  Derivative : Derivative
  Derivative1 : Derivative
  Derivative2 : Derivative
  Gain : Gain  Gain=1/J_MS
  Gain1 : Gain  Gain=Rs_MS/(J_MS*Lq_MS)
  Gain2 : Gain  Gain=gamq
  Product : Product
  Product1 : Product
  alpha_0_wMS : Subsystem
  alpha_1_wMS : Subsystem
  Phi : Outport
  tag scope: D_wMS_des=global
  wires:
  wr_deseada/1 -> Product1/1, Derivative/1
  Derivative/1 -> Product/1, [D_wMS_des], Derivative1/1
  TLmsin/1 -> Derivative2/1, Gain1/1
  Derivative1/1 -> Add/1
  Product/1 -> Add/2
  Product1/1 -> Add/3
  Add/1 -> Gain2/1
  Gain2/1 -> Phi/1
  Add1/1 -> Add/4  "psi_MS"
  Gain/1 -> Add1/1
  Gain1/1 -> Add1/2
  Derivative2/1 -> Gain/1
  [alpha1a_wMS] -> Product/2
  [alpha0a_wMS] -> Product1/2

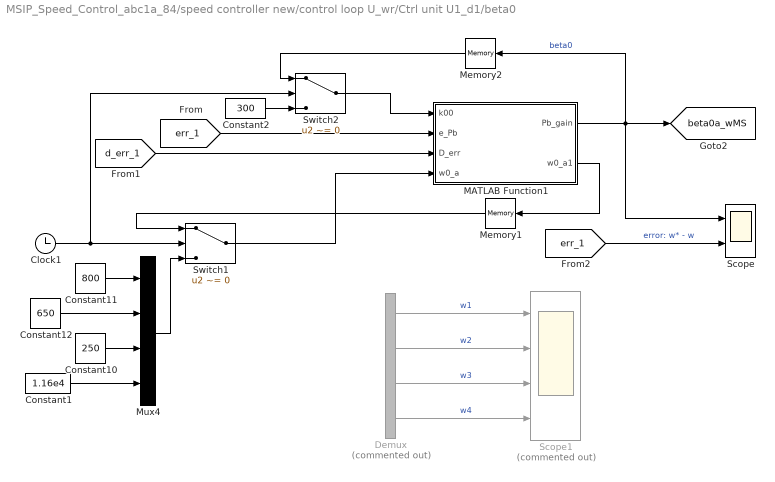
== system MSIP_Speed_Control_abc1a_84/speed controller new/control loop U_wr/Ctrl unit U1_d1/beta0 ==
  Clock1 : Clock
  Constant1 : Constant  Value=1.16e4
  Constant10 : Constant  Value=250
  Constant11 : Constant  Value=800
  Constant12 : Constant  Value=650
  Constant2 : Constant  Value=300
  Demux : Demux  Commented=on
  MATLAB Function1 : MATLAB Function  TreatAsAtomicUnit=on
  Memory1 : Memory
  Memory2 : Memory
  Mux4 : Mux
  Scope : Scope  NumInputPorts=2
      settings: ActiveDisplayYMinimum=-36930.77862  ActiveDisplayYMaximum=335377.00762
  Scope1 : Scope  Commented=on  NumInputPorts=4
      settings: ActiveDisplayYMinimum=-442.05631  ActiveDisplayYMaximum=11978.50681  DataLoggingVariableName=ScopeData2
  Switch1 : Switch  Criteria=u2 ~= 0  SaturateOnIntegerOverflow=off  InputSameDT=off
  Switch2 : Switch  Criteria=u2 ~= 0  SaturateOnIntegerOverflow=off  InputSameDT=off
  tag scope: beta0a_wMS=global
  wires:
  [err_1] -> Scope/2  "error: w* - w"
  Constant12/1 -> Mux4/2
  [err_1] -> MATLAB Function1/2(e_Pb)
  Constant10/1 -> Mux4/3
  Memory1/1 -> Switch1/1
  MATLAB Function1/1(Pb_gain) -> Memory2/1, Scope/1, [beta0a_wMS]  "beta0"
  Mux4/1 -> Switch1/3
  Clock1/1 -> Switch2/2, Switch1/2
  MATLAB Function1/2(w0_a1) -> Memory1/1
  Constant11/1 -> Mux4/1
  [d_err_1] -> MATLAB Function1/3(D_err)
  Constant1/1 -> Mux4/4
  Switch1/1 -> MATLAB Function1/4(w0_a)
  Memory2/1 -> Switch2/1
  Constant2/1 -> Switch2/3
  Switch2/1 -> MATLAB Function1/1(k00)
  Demux/3 -> Scope1/3  "w3"
  Demux/2 -> Scope1/2  "w2"
  Demux/1 -> Scope1/1  "w1"
  Demux/4 -> Scope1/4  "w4"

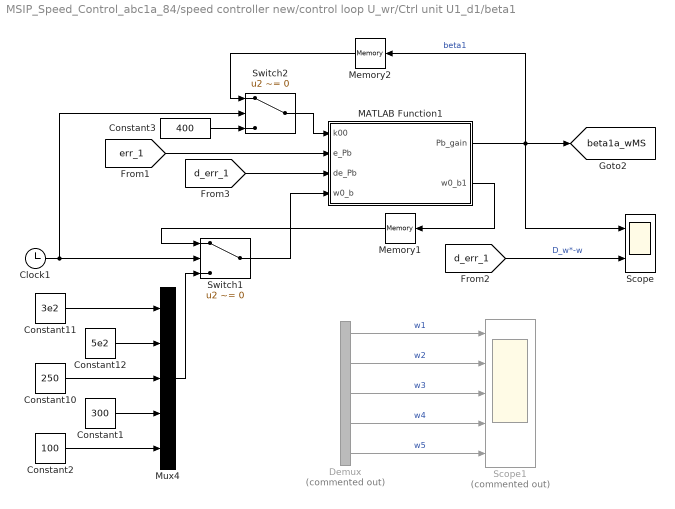
== system MSIP_Speed_Control_abc1a_84/speed controller new/control loop U_wr/Ctrl unit U1_d1/beta1 ==
  Clock1 : Clock
  Constant1 : Constant  Value=300
  Constant10 : Constant  Value=250
  Constant11 : Constant  Value=3e2
  Constant12 : Constant  Value=5e2
  Constant2 : Constant  Value=100
  Constant3 : Constant  Value=400
  Demux : Demux  Commented=on  Outputs=5
  MATLAB Function1 : MATLAB Function  TreatAsAtomicUnit=on
  Memory1 : Memory
  Memory2 : Memory
  Mux4 : Mux  Inputs=5
  Scope : Scope  NumInputPorts=2
      settings: ActiveDisplayYMinimum=211.34021  ActiveDisplayYMaximum=2097.93807
  Scope1 : Scope  Commented=on  NumInputPorts=5
      settings: ActiveDisplayYMinimum=299.4945  ActiveDisplayYMaximum=304.54948
  Switch1 : Switch  Criteria=u2 ~= 0  SaturateOnIntegerOverflow=off  InputSameDT=off
  Switch2 : Switch  Criteria=u2 ~= 0  SaturateOnIntegerOverflow=off  InputSameDT=off
  tag scope: beta1a_wMS=global
  wires:
  [d_err_1] -> Scope/2  "D_w*-w"
  Constant12/1 -> Mux4/2
  Constant10/1 -> Mux4/3
  Memory1/1 -> Switch1/1
  MATLAB Function1/1(Pb_gain) -> Memory2/1, Scope/1, [beta1a_wMS]  "beta1"
  Mux4/1 -> Switch1/3
  Switch1/1 -> MATLAB Function1/4(w0_b)
  Clock1/1 -> Switch2/2, Switch1/2
  MATLAB Function1/2(w0_b1) -> Memory1/1
  Constant11/1 -> Mux4/1
  Constant1/1 -> Mux4/4
  [err_1] -> MATLAB Function1/2(e_Pb)
  [d_err_1] -> MATLAB Function1/3(de_Pb)
  Constant2/1 -> Mux4/5
  Demux/1 -> Scope1/1  "w1"
  Demux/2 -> Scope1/2  "w2"
  Demux/3 -> Scope1/3  "w3"
  Demux/4 -> Scope1/4  "w4"
  Demux/5 -> Scope1/5  "w5"
  Switch2/1 -> MATLAB Function1/1(k00)
  Memory2/1 -> Switch2/1
  Constant3/1 -> Switch2/3

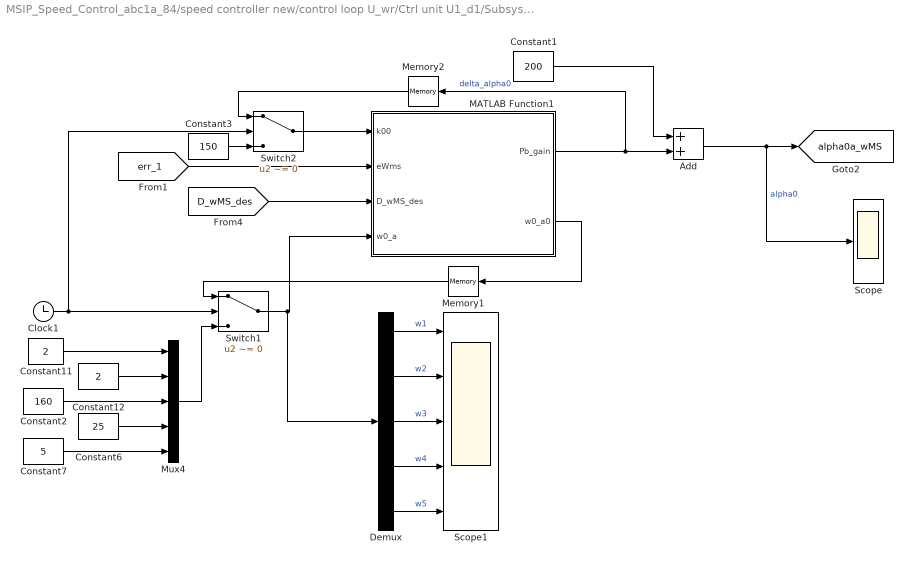
== system MSIP_Speed_Control_abc1a_84/speed controller new/control loop U_wr/Ctrl unit U1_d1/Subsystem/alpha_0_wMS ==
  Add : Sum
  Clock1 : Clock
  Constant1 : Constant  Value=200
  Constant11 : Constant  Value=2
  Constant12 : Constant  Value=2
  Constant2 : Constant  Value=160
  Constant3 : Constant  Value=150
  Constant6 : Constant  Value=25
  Constant7 : Constant  Value=5
  Demux : Demux  Outputs=5
  MATLAB Function1 : MATLAB Function  TreatAsAtomicUnit=on
  Memory1 : Memory
  Memory2 : Memory
  Mux4 : Mux  Inputs=5
  Scope : Scope
      settings: ActiveDisplayYMinimum=334.23855  ActiveDisplayYMaximum=357.01533
  Scope1 : Scope  NumInputPorts=5
      settings: ActiveDisplayYMinimum=1.88699  ActiveDisplayYMaximum=3.01705
  Switch1 : Switch  Criteria=u2 ~= 0  SaturateOnIntegerOverflow=off  InputSameDT=off
  Switch2 : Switch  Criteria=u2 ~= 0  SaturateOnIntegerOverflow=off  InputSameDT=off
  tag scope: alpha0a_wMS=global
  wires:
  Constant11/1 -> Mux4/1
  MATLAB Function1/2(w0_a0) -> Memory1/1
  Clock1/1 -> Switch2/2, Switch1/2
  Switch1/1 -> Demux/1, MATLAB Function1/4(w0_a)
  Mux4/1 -> Switch1/3
  Memory1/1 -> Switch1/1
  Constant12/1 -> Mux4/2
  [err_1] -> MATLAB Function1/2(eWms)
  Demux/1 -> Scope1/1  "w1"
  Demux/2 -> Scope1/2  "w2"
  [D_wMS_des] -> MATLAB Function1/3(D_wMS_des)
  Constant1/1 -> Add/1
  MATLAB Function1/1(Pb_gain) -> Memory2/1, Add/2  "delta_alpha0"
  Constant2/1 -> Mux4/3
  Demux/3 -> Scope1/3  "w3"
  Constant6/1 -> Mux4/4
  Demux/4 -> Scope1/4  "w4"
  Demux/5 -> Scope1/5  "w5"
  Constant7/1 -> Mux4/5
  Switch2/1 -> MATLAB Function1/1(k00)
  Constant3/1 -> Switch2/3
  Memory2/1 -> Switch2/1
  Add/1 -> [alpha0a_wMS], Scope/1  "alpha0"

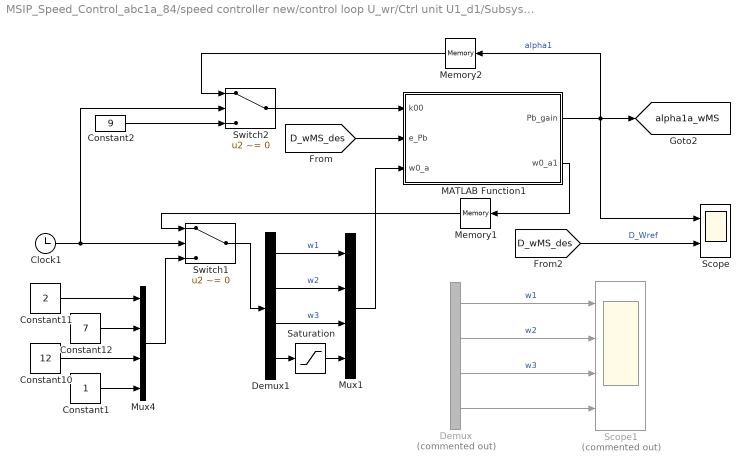
== system MSIP_Speed_Control_abc1a_84/speed controller new/control loop U_wr/Ctrl unit U1_d1/Subsystem/alpha_1_wMS ==
  Clock1 : Clock
  Constant1 : Constant
  Constant10 : Constant  Value=12
  Constant11 : Constant  Value=2
  Constant12 : Constant  Value=7
  Constant2 : Constant  Value=9
  Demux : Demux  Commented=on
  Demux1 : Demux
  MATLAB Function1 : MATLAB Function  TreatAsAtomicUnit=on
  Memory1 : Memory
  Memory2 : Memory
  Mux1 : Mux
  Mux4 : Mux
  Saturation : Saturate  UpperLimit=50  LowerLimit=-50
  Scope : Scope  NumInputPorts=2
      settings: ActiveDisplayYMinimum=-43.88992  ActiveDisplayYMaximum=26.0794
  Scope1 : Scope  Commented=on  NumInputPorts=4
      settings: ActiveDisplayYMinimum=1.99494  ActiveDisplayYMaximum=2.04551  DataLoggingVariableName=ScopeData3
  Switch1 : Switch  Criteria=u2 ~= 0  SaturateOnIntegerOverflow=off  InputSameDT=off
  Switch2 : Switch  Criteria=u2 ~= 0  SaturateOnIntegerOverflow=off  InputSameDT=off
  tag scope: alpha1a_wMS=global
  wires:
  [D_wMS_des] -> Scope/2  "D_Wref"
  Constant12/1 -> Mux4/2
  [D_wMS_des] -> MATLAB Function1/2(e_Pb)
  Constant10/1 -> Mux4/3
  Memory1/1 -> Switch1/1
  MATLAB Function1/1(Pb_gain) -> Memory2/1, Scope/1, [alpha1a_wMS]  "alpha1"
  Clock1/1 -> Switch2/2, Switch1/2
  MATLAB Function1/2(w0_a1) -> Memory1/1
  Constant11/1 -> Mux4/1
  Demux/2 -> Scope1/2  "w2"
  Demux/1 -> Scope1/1  "w1"
  Demux/3 -> Scope1/3  "w3"
  Switch2/1 -> MATLAB Function1/1(k00)
  Mux4/1 -> Switch1/3
  Constant2/1 -> Switch2/3
  Memory2/1 -> Switch2/1
  Demux/4 -> Scope1/4
  Constant1/1 -> Mux4/4
  Switch1/1 -> Demux1/1
  Demux1/1 -> Mux1/1  "w1"
  Demux1/2 -> Mux1/2  "w2"
  Demux1/3 -> Mux1/3  "w3"
  Mux1/1 -> MATLAB Function1/3(w0_a)
  Demux1/4 -> Saturation/1
  Saturation/1 -> Mux1/4

== matlab function MSIP_Speed_Control_abc1a_84/b)VSC_84/PLL/Module ==
  data: u input; y output
function y = fcn(u)
if (and(u(1)==0,u(2)==0))
    y=1;
else
    y = sqrt(u(1)*u(1)+u(2)*u(2));
end

== matlab function MSIP_Speed_Control_abc1a_84/3 Nm/TL2 ==
  data: t input; T_load2 output
function T_load2 = Tload2(t)
    
t1 = 85;   %  " initial and final instants of rest-to-rest
t2 = 90;

delt = t2-t1;
tdif = abs(t-t1) ;

% " initial and final values 
z1in = 0;
z1f  = -25;

%z1f  = dta0;

z1dif = z1f-z1in;

tau=(tdif/delt);
tau2=tau*tau;
tau3=tau*tau2;
tau4=tau*tau3;
tau5=tau*tau4;
tau6=tau*tau5;
tau7=tau*tau6;
tau8=tau*tau7;
tau9=tau*tau8;

r1=12870;
r2=91520;
r3=288288;
r4=524160;
r5=600600;
r6=443520;
r7=205920;
r8=54912;
r9=6435;

z1st1 = z1in;
fr    = r1-r2*tau+r3*tau2-r4*tau3+r5*tau4-r6*tau5+r7*tau6-r8*tau7+r9*tau8;
z1stt = z1in+z1dif*tau8*fr;
z1st2 = z1f;


    if t<t1
         T_load2     = z1st1; 
    elseif t<t2
         T_load2     = z1stt; 
    else
         T_load2     = z1st2; 
    end

== matlab function MSIP_Speed_Control_abc1a_84/3 Nm/TL3 ==
  data: t input; T_load3 output
function T_load3 = Tload3(t)
    
t1 = 125;   %  " initial and final instants of rest-to-rest
t2 = 135;

delt = t2-t1;
tdif = abs(t-t1) ;

% " initial and final values 
z1in = 0;
z1f  = 34;

%z1f  = dta0;

z1dif = z1f-z1in;

tau=(tdif/delt);
tau2=tau*tau;
tau3=tau*tau2;
tau4=tau*tau3;
tau5=tau*tau4;
tau6=tau*tau5;
tau7=tau*tau6;
tau8=tau*tau7;
tau9=tau*tau8;

r1=12870;
r2=91520;
r3=288288;
r4=524160;
r5=600600;
r6=443520;
r7=205920;
r8=54912;
r9=6435;

z1st1 = z1in;
fr    = r1-r2*tau+r3*tau2-r4*tau3+r5*tau4-r6*tau5+r7*tau6-r8*tau7+r9*tau8;
z1stt = z1in+z1dif*tau8*fr;
z1st2 = z1f;


    if t<t1
         T_load3     = z1st1; 
    elseif t<t2
         T_load3     = z1stt; 
    else
         T_load3     = z1st2; 
    end

== matlab function MSIP_Speed_Control_abc1a_84/b)VSC_84/PULSES_YY/MATLAB Function ==
  data: u input; s1 output; s2 output; s3 output; s4 output; s5 output; s6 output
function [s1,s2,s3,s4,s5,s6]= fcn(u)
    if  u>5*1.0472 %pi/3=1.0472
        s1=0;s2=0;s3=0;s4=1;s5=1;s6=1;
    elseif u>4*1.0472
        s1=0;s2=0;s3=1;s4=1;s5=1;s6=0;
    elseif u>pi
        s1=0;s2=1;s3=1;s4=1;s5=0;s6=0;        
    elseif u>2*1.0472
        s1=1;s2=1;s3=1;s4=0;s5=0;s6=0;
    elseif u>(1.0472)
        s1=1;s2=1;s3=0;s4=0;s5=0;s6=1;
    elseif u>0
        s1=1;s2=0;s3=0;s4=0;s5=1;s6=1;
    else
        s1=0;s2=0;s3=0;s4=0;s5=0;s6=0;
    
end

== matlab function MSIP_Speed_Control_abc1a_84/speed controller new/control loop U_wr/Ctrl unit U1_d1/Subsystem/alpha_0_wMS/MATLAB Function1 ==
  data: k00 input; eWms input; D_wMS_des input; Pb_gain output; w0_a input; w0_a0 output
function [Pb_gain,w0_a0] = fcn_gainalpha0(k00,eWms,D_wMS_des,w0_a)

D_eN = D_wMS_des;
    if abs(eWms) > 0.01 %0.05
        etaN = 5e-4; %5e-4;
         aNNa0        = [fun_base_1var_3orden_1a(D_eN)...
                         fun_base_1var_3orden_2a(D_eN)...
                         fun_base_1var_3orden_3a(eWms)...
                         fun_base_1var_3orden_4a(eWms)...
                         fun_base_1var_3orden_4a(-eWms)];
         
         B01          =  norm(aNNa0,2)^2;
        if B01<=0
            B0 = 1e-6;
        else
            B0 = B01;
        end
         w0_a0        =  w0_a + etaN*(eWms/B0)*(aNNa0.');
         Pb_gain      =  aNNa0*w0_a0;
    else
         w0_a0        =  w0_a;
         Pb_gain      =  k00;
    end

== matlab function MSIP_Speed_Control_abc1a_84/speed controller new/control loop U_wr/Ctrl unit U1_d1/Subsystem/alpha_1_wMS/MATLAB Function1 ==
  data: k00 input; e_Pb input; Pb_gain output; w0_a input; w0_a1 output
function [Pb_gain,w0_a1] = fcn_gainalpha1(k00,e_Pb,w0_a)

eN   = e_Pb;
    
    if abs(eN) > 10 %0.5
        etaN = 1e-5; %1e-6;
        aNNa0        = [fun_base_1var_3orden(eN)...
                        fun_base_1var_3orden_a(eN)...
                        fun_base_1var_3orden_a(eN)...
                        fun_base_1var_3orden_b(eN)];
        B01          =  norm(aNNa0,2)^2;
        if B01<=0
            B0 = 1e-6;
        else
            B0 = B01;
        end
        w0_a1        =  w0_a + etaN*(eN/B0)*(aNNa0.');
        Pb_gain      =  aNNa0*w0_a1;
    else
        w0_a1        =  w0_a;
        Pb_gain      =  k00;
    end

== matlab function MSIP_Speed_Control_abc1a_84/speed controller new/control loop U_wr/Ctrl unit U1_d1/beta0/MATLAB Function1 ==
  data: k00 input; e_Pb input; D_err input; Pb_gain output; w0_a input; w0_a1 output
function [Pb_gain,w0_a1] = fcn_gainBTA0(k00,e_Pb,D_err,w0_a)

eN   = e_Pb;

    if abs(eN) > 0.005 %0.05
            etaN = 15; %10;
            aNNa0        = [fun_base_1var_3orden(eN)...
                            fun_base_1var_3orden_a(eN)...
                            fun_base_1var_3orden_b(eN)...
                            fun_base_1var_3orden(D_err)];
            B01          =  norm(aNNa0,2)^2;
            if B01<=0
                B0 = 1e-6;
            else
                B0 = B01;
            end
             w0_a1        =  w0_a + etaN*(eN/B0)*(aNNa0.');
             Pb_gain = aNNa0*w0_a1;
    else
        w0_a1        =  w0_a;
        Pb_gain      =  k00;
    end

== matlab function MSIP_Speed_Control_abc1a_84/speed controller new/control loop U_wr/Ctrl unit U1_d1/beta1/MATLAB Function1 ==
  data: k00 input; e_Pb input; de_Pb input; Pb_gain output; w0_b input; w0_b1 output
function [Pb_gain,w0_b1] = fcn_gainBTA1(k00,e_Pb,de_Pb,w0_b)

eN1   = e_Pb;
eN2   = de_Pb;
    
    if abs(eN1) > 0.06 %0.05
        etaN = 0.1; %0.05;
        aNNa0        = [fun_base_1var_3orden(eN1)...
                        fun_base_1var_3orden_a(eN2)...
                        fun_base_1var_3orden_b(eN1)...
                        fun_base_1var_3orden_b(eN2)...
                        fun_base_1var_3orden_a(eN1)];
        B01          =  norm(aNNa0,2)^2;
        if B01<=0
            B0 = 1e-6;
        else
            B0 = B01;
        end
        w0_b1        =  w0_b + etaN*(eN1/B0)*(aNNa0.');
        Pb_gain      = aNNa0*w0_b1;
    else
        w0_b1        =  w0_b;
        Pb_gain      =  k00;
    end
